simulink model "positionpid_rtsim"  (R2022b)
settings: Solver=FixedStepAuto  StartTime=0.0  StopTime=5  FixedStep=0.001  RelTol=1e-3
values from neighbouring files (symbols this model uses):
  Kw = 1 / Tw    [pid_calibration.m]    (also in positionpid.m)
undefined symbols (not defined in the file or in its folder): National_Instruments, PCIe, PID, sens
libraries: sldrtlib x3
settings Model: SimulationMode=external  ExtModeTrigDuration=100001  ExtModeTrigDurationFloating=100001  Creator=lucas  LastModifiedBy=gottardofi
settings DataIOCC: ReturnWorkspaceOutputs=off
settings HardwareCC: ProdBitPerLong=64  ProdHWDeviceType=Intel->x86-64 (Linux 64)
settings RTWCC: Description=Simulink Desktop Real-Time  SystemTargetFile=sldrt.tlc  TemplateMakefile=sldrt.tmf  RTWCompilerOptimization=on
settings CodeAppCC: MaxIdLength=95
settings SimulinkDesktopRealTimeCC: TargetLibSuffix=_sldrt.a  TargetPreCompLibLocation=C:\Program Files\MATLAB\R2022b\toolbox\sldrt\lib\win64

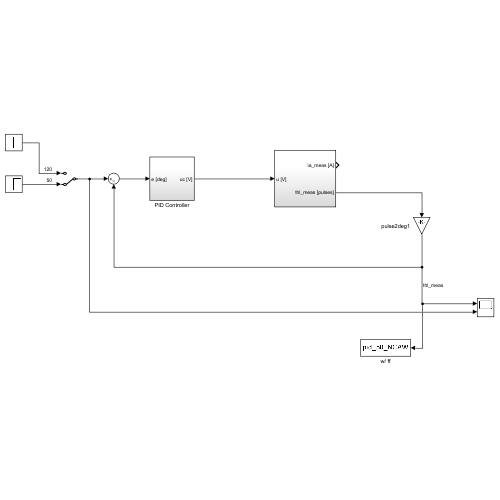
[thumbnail: Simulink's stored preview of the top-level diagram]
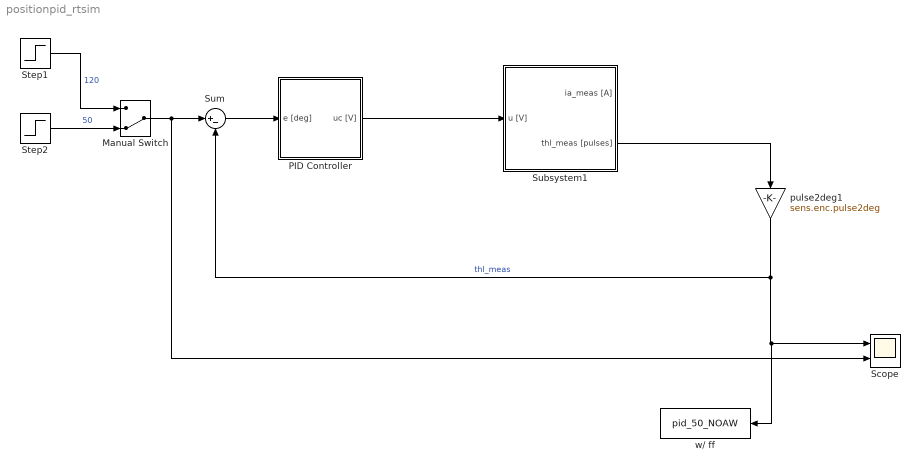
== system positionpid_rtsim ==
  Manual Switch : ManualSwitch  CurrentSetting=0
  PID Controller : Subsystem
  Scope : Scope  NumInputPorts=2
  Step1 : Step  After=120  SampleTime=0
  Step2 : Step  After=50  SampleTime=0
  Subsystem1 : Subsystem
  Sum : Sum  Inputs=|+-
  pulse2deg1 : Gain  Gain=sens.enc.pulse2deg
  w/ ff : ToWorkspace  VariableName=pid_50_NOAW  SaveFormat=Structure With Time  SampleTime=-1
  wires:
  pulse2deg1/1 -> w/ ff/1, Scope/1, Sum/2  "thl_meas"
  Sum/1 -> PID Controller/1(e [deg])
  PID Controller/1(uc [V]) -> Subsystem1/1(u [V])
  Subsystem1/2(thl_meas [pulses]) -> pulse2deg1/1
  Manual Switch/1 -> Scope/2, Sum/1
  Step1/1 -> Manual Switch/1  "120"
  Step2/1 -> Manual Switch/2  "50"

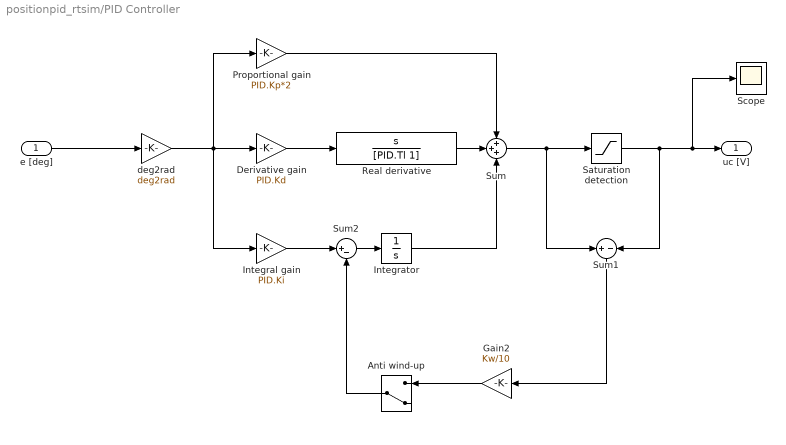
== system positionpid_rtsim/PID Controller ==
  e [deg] : Inport
  Anti wind-up : ManualSwitch  CurrentSetting=0
  Derivative gain : Gain  Gain=PID.Kd
  Gain2 : Gain  Gain=Kw/10
  Integral gain : Gain  Gain=PID.Ki
  Integrator : Integrator
  Proportional gain : Gain  Gain=PID.Kp*2
  Real derivative : TransferFcn  Numerator=[1, 0]  Denominator=[PID.Tl 1]
  Saturation detection : Saturate  UpperLimit=10  LowerLimit=-10
  Scope : Scope
  Sum : Sum  Inputs=+++
  Sum1 : Sum  Inputs=+|-
  Sum2 : Sum  Inputs=|+-
  deg2rad : Gain  Gain=deg2rad
  uc [V] : Outport
  wires:
  Real derivative/1 -> Sum/2
  Derivative gain/1 -> Real derivative/1
  Sum2/1 -> Integrator/1
  deg2rad/1 -> Integral gain/1, Derivative gain/1, Proportional gain/1
  Sum/1 -> Sum1/1, Saturation detection/1
  Anti wind-up/1 -> Sum2/2
  Integrator/1 -> Sum/3
  Gain2/1 -> Anti wind-up/1
  Proportional gain/1 -> Sum/1
  Integral gain/1 -> Sum2/1
  Sum1/1 -> Gain2/1
  e [deg]/1 -> deg2rad/1
  Saturation detection/1 -> Scope/1, uc [V]/1, Sum1/2

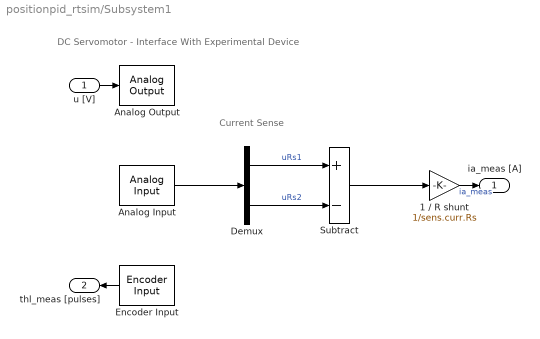
== system positionpid_rtsim/Subsystem1 ==
  note: DC Servomotor - Interface With Experimental Device
  note: Current Sense
  u [V] : Inport
  1 / R shunt : Gain  Gain=1/sens.curr.Rs
  Analog Input : sldrtlib/Analog Input  SampleTime=-1  MaxMissedTicks=10  ShowMissedTicks=off  YieldWhenWaiting=off  DrvName=National_Instruments/PCIe-6321  DrvAddress=4294967295  DrvOptions=[0 0 0 2 0 0 0]  Channels=[1, 2]  RangeMode=1  VoltRange=1  DataType=1
      settings: AttributesFormatString=National Instruments\nPCIe-6321 [auto]
  Analog Output : sldrtlib/Analog Output  SampleTime=-1  MaxMissedTicks=10  ShowMissedTicks=off  YieldWhenWaiting=off  DrvName=National_Instruments/PCIe-6321  DrvAddress=4294967295  DrvOptions=[0 0 0 2 0 0 0]  Channels=1  RangeMode=1  VoltRange=1  InitialValue=0  FinalValue=0
      settings: AttributesFormatString=National Instruments\nPCIe-6321 [auto]
  Demux : Demux  Outputs=2
  Encoder Input : sldrtlib/Encoder Input  SampleTime=-1  MaxMissedTicks=10  ShowMissedTicks=off  YieldWhenWaiting=off  DrvName=National_Instruments/PCIe-6321  DrvAddress=4294967295  DrvOptions=[0 0 0 2 0 0 0]  Channels=1  QuadMode=3  IndexPulse=1  InputFilter=Inf  DataType=1
      settings: AttributesFormatString=National Instruments\nPCIe-6321 [auto]
  Subtract : Sum  Inputs=+-
  ia_meas [A] : Outport
  thl_meas [pulses] : Outport  Port=2
  wires:
  u [V]/1 -> Analog Output/1
  Subtract/1 -> 1 / R shunt/1
  Demux/2 -> Subtract/2  "uRs2"
  Encoder Input/1 -> thl_meas [pulses]/1
  1 / R shunt/1 -> ia_meas [A]/1  "ia_meas"
  Analog Input/1 -> Demux/1
  Demux/1 -> Subtract/1  "uRs1"
